simulink model "pacificpower360amxt"  (R2018b)
settings: Solver=VariableStepAuto  StartTime=0.0  StopTime=10  FixedStep=0.001  RelTol=1e-3
libraries: fl_lib x25, nesl_utility x19, powerlib_meascontrol x12, simulink x12
settings Model: Creator=opal  LastModifiedBy=mne4
settings SFSimCC: SimUseLocalCustomCode=off
settings RTWCC: RTWUseLocalCustomCode=off
settings CodeAppCC: StateflowObjectComments=on
settings SimscapeCC: SimscapeNormalizeSystem=off

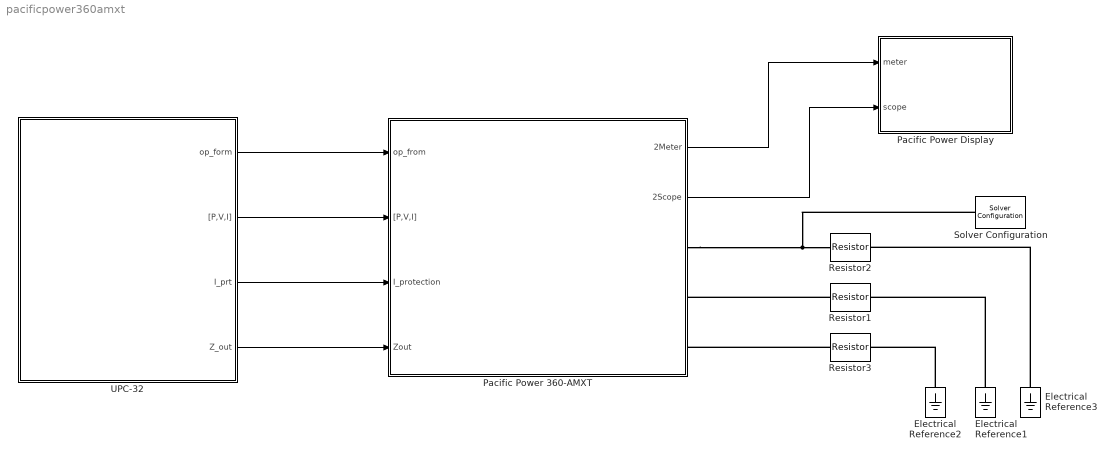
== system pacificpower360amxt ==
  Electrical Reference1 : fl_lib/Electrical/Electrical Elements/Electrical Reference
  Electrical Reference2 : fl_lib/Electrical/Electrical Elements/Electrical Reference
  Electrical Reference3 : fl_lib/Electrical/Electrical Elements/Electrical Reference
  Pacific Power 360-AMXT : Subsystem  mask{p_switch=1, VslewAC=5.000e+05, FslewAC=500.0, VslewDC=20000.0, IslewDC=1.000e+05, PslewDC=1.000e+06}
      mask prompts: p_switch "Enter 1 to turn ON, 0 to turn OFF NHR 9410"
      mask DialogControl DescTextVar Prompt: Pacific Power 360-AMXT (transformer coupled)
      mask DialogControl Container3 Prompt: Slew Rates
      mask DialogControl Control2 Prompt: AC Voltage slew rate [0-500000V/s]:
      mask DialogControl f Prompt: Frequency slew rate [0-500 /s]
      mask DialogControl Control3 Prompt: DC Voltage slew rate [0-20000V/s]:
      mask DialogControl Control4 Prompt: DC current slew rate [0-100000A/s]:
      mask DialogControl Control5 Prompt: DC power slew rate [0-1000000W/s]:
      mask Display: image('pacificpower360AMXT.png');
  Pacific Power Display : Subsystem
  Resistor1 : fl_lib/Electrical/Electrical Elements/Resistor  R=1.66 Ohm  i_specify=off  i_priority=None  i=0 A  i_nominal_specify=off  i_nominal_unit=A  i_nominal_value=1  v_specify=off  v_priority=None  v=0 V  v_nominal_specify=off  v_nominal_unit=V  v_nominal_value=1
  Resistor2 : fl_lib/Electrical/Electrical Elements/Resistor  R=1.66 Ohm  i_specify=off  i_priority=None  i=0 A  i_nominal_specify=off  i_nominal_unit=A  i_nominal_value=1  v_specify=off  v_priority=None  v=0 V  v_nominal_specify=off  v_nominal_unit=V  v_nominal_value=1
  Resistor3 : fl_lib/Electrical/Electrical Elements/Resistor  R=1.66 Ohm  i_specify=off  i_priority=None  i=0 A  i_nominal_specify=off  i_nominal_unit=A  i_nominal_value=1  v_specify=off  v_priority=None  v=0 V  v_nominal_specify=off  v_nominal_unit=V  v_nominal_value=1
  Solver Configuration : nesl_utility/Solver Configuration  PhysicalDomain=network_engine_domain  SubClassName=solver  LeftPortType=input  RightPortType=generic  Tones=[]  Harmonics=[]  SimulateNoise=off  Profile=off  UseLocalSampling=off  EnableSwitchedLinearOptims=on  FrequencyDomain=off  UseCCode=off  RelTol=0.001  AbsTol=1e-06  MinStep=1e-09  ToWorkspace=off  RevertToSquareIcSolve=off  NumHomotopyIterations=100  PhasorMode=off  PhasorModeNumHarmonics=1  DoDC=off  ResidualTolerance=1e-09  UseLocalSolver=on  LocalSolverChoice=NE_BACKWARD_EULER_ADVANCER  LocalSolverSampleTime=0.001  DoFixedCost=on  MaxNonlinIter=3  MaxModeIter=2  LinearAlgebra=Sparse  EquationFormulation=NE_TIME_EF  DelaysMemoryBudget=1024  AutomaticFiltering=off  FilteringTimeConstant=0.001  PartitionStorageMethod=AS_NEEDED  PartitionMemoryBudget=1024
  UPC-32 : Subsystem  mask{f=60, sel=1, form_sel=1, Vm11=100, Im11=10, Vm12=100, Im12=10, Vm13a=100, Vm13b=100, Vm13c=100, Ph13b=120, Ph13c=240, Im13=10, Vm21=100, Im21=0, Vm22=100, Im22=0, Vm23a=100, Vm23b=100, Vm23c=100, Ph23b=120, Ph23c=240, Im23=10, Zout=10, Iprt=0, Iprtlim=0, Tiprt=0}
      mask prompts: sel "Enter "1" for direct coupling, or "2" for transformner (2.0:1) coupling:"; form_sel "Enter "1" for 1-phase (Form-1), "2" for 2-phase (Form-2), "3" for 3-phase (Form-3):"; Iprt "Current protection (1: ON, 0: OFF):"; Iprtlim "Current protection limit:"; Tiprt "Current protection time:"
      mask DialogControl DescTextVar Prompt: UPC-32 (Universal Programmable Controller)
      mask DialogControl Control30 Prompt: Frequency (Hz) [20-5000Hz]:
      mask DialogControl Container12 Prompt: Direct Coupling
      mask DialogControl Container67 Prompt: Expand selected form and enter input parameters
      mask DialogControl Container66 Prompt: Form-1: 1-phase AC
      mask DialogControl Control311 Prompt: Voltage limit (Vrms l-n) [0-135V]:
      mask DialogControl Control29 Prompt: Current limit (Irms/phase) [0-48A]:
      mask DialogControl Container68 Prompt: Form-2: 2-phase AC
      mask DialogControl Control3_copy Prompt: Voltage limit (Vrms l-l) [0-270V]:
      mask DialogControl Control36 Prompt: Current limit (Irms/phase) [0-16A]:
      mask DialogControl Container69 Prompt: Form-3: 3-phase AC
      mask DialogControl Control331 Prompt: Voltage limit (Vrms l-n) [0-135V], Phase A:
      mask DialogControl Control31 Prompt: Voltage limit (Vrms l-n) [0-135V], Phase B:
      mask DialogControl Control32 Prompt: Voltage limit (Vrms l-n) [0-135V], Phase C:
      mask DialogControl Control33 Prompt: Phase A angle (degrees): 0
      mask DialogControl Control34 Prompt: Phase B angle (degrees):
      mask DialogControl Control35 Prompt: Phase C angle (degrees):
      mask DialogControl Control37 Prompt: Current limit (Irms/phase) [0-16A]:
      mask DialogControl Container12_copy Prompt: Transformer Coupling
      mask DialogControl Container67_copy Prompt: Expand selected form and enter input parameters
      mask DialogControl Container66_copy Prompt: Form-1: 1-phase AC
      mask DialogControl Control311_copy Prompt: Voltage limit (Vrms l-n) [0-273V]:
      mask DialogControl Control29_copy Prompt: Current limit (Irms/phase) [0-24A]:
      mask DialogControl Container68_copy Prompt: Form-2: 2-phase AC
      mask DialogControl Control3_copy_copy Prompt: Voltage limit (Vrms l-l) [0-546V]:
      mask DialogControl Control36_copy Prompt: Current limit (Irms/phase) [0-8A]:
      mask DialogControl Container69_copy Prompt: Form-3: 3-phase AC
      mask DialogControl Control331_copy Prompt: Voltage limit (Vrms l-n) [0-273V], Phase A:
      mask DialogControl Control31_copy Prompt: Voltage limit (Vrms l-n) [0-273V], Phase B:
      mask DialogControl Control32_copy Prompt: Voltage limit (Vrms l-n) [0-273V], Phase C:
      mask DialogControl Control33_copy Prompt: Phase A angle (degrees): 0
      mask DialogControl Control34_copy Prompt: Phase B angle (degrees):
      mask DialogControl Control35_copy Prompt: Phase C angle (degrees):
      mask DialogControl Control37_copy Prompt: Current limit (Irms/phase) [0-8A]:
      mask DialogControl Control27 Prompt: Output impedance
      mask Display: image('upc32.png');
  wires:
  UPC-32/1(op_form) -> Pacific Power 360-AMXT/1(op_from)
  UPC-32/2("[P,V,I]") -> Pacific Power 360-AMXT/2("[P,V,I]")
  UPC-32/3(I_prt) -> Pacific Power 360-AMXT/3(I_protection)
  UPC-32/4(Z_out) -> Pacific Power 360-AMXT/4(Zout)
  Pacific Power 360-AMXT/1(2Meter) -> Pacific Power Display/1(meter)
  Pacific Power 360-AMXT/2(2Scope) -> Pacific Power Display/2(scope)
  connections:
  Pacific Power 360-AMXT/RConn1 -- Solver Configuration/RConn1 -- Resistor2/LConn1
  Electrical Reference3/LConn1 -- Resistor2/RConn1
  Resistor1/LConn1 -- Pacific Power 360-AMXT/RConn2
  Resistor3/LConn1 -- Pacific Power 360-AMXT/RConn3
  Electrical Reference2/LConn1 -- Resistor3/RConn1
  Electrical Reference1/LConn1 -- Resistor1/RConn1

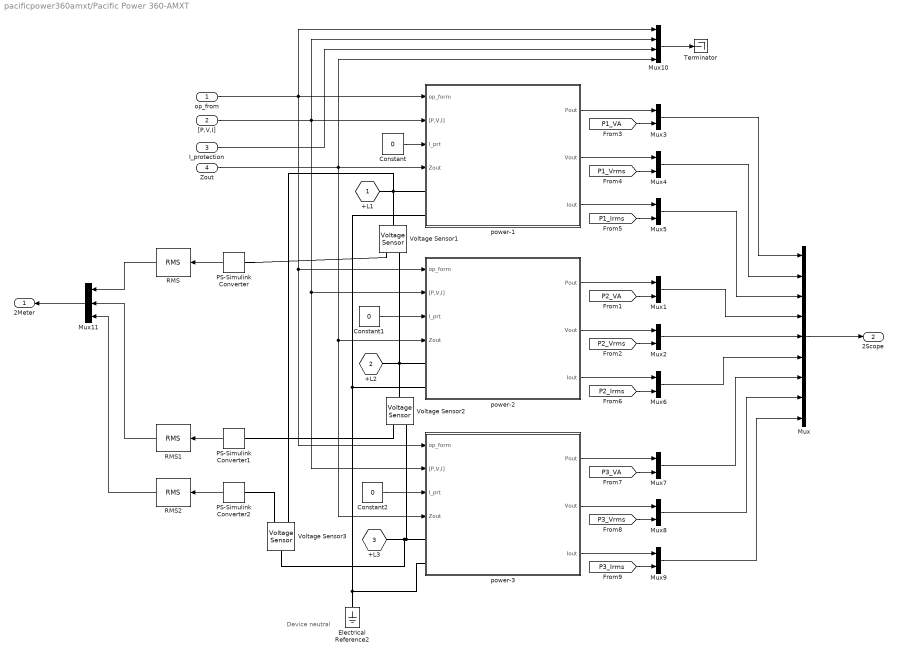
== system pacificpower360amxt/Pacific Power 360-AMXT ==
  note: Device neutral
  op_from : Inport
  "[P,V,I]" : Inport  Port=2
  I_protection : Inport  Port=3
  Zout : Inport  Port=4
  Constant : Constant  Value=0
  Constant1 : Constant  Value=0
  Constant2 : Constant  Value=0
  Electrical Reference2 : fl_lib/Electrical/Electrical Elements/Electrical Reference
  Mux : Mux  Inputs=9
  Mux{1..9} (9 alike) : Mux  Inputs=2
  Mux10 : Mux
  Mux11 : Mux  Inputs=3
  PS-Simulink Converter : nesl_utility/PS-Simulink Converter  PhysicalDomain=network_engine_domain  SubClassName=ps_output  LeftPortType=input  RightPortType=output  PseudoPeriodic=off  Frequencies=[]  Unit=1  AffineConversion=off
  PS-Simulink Converter1 : nesl_utility/PS-Simulink Converter  PhysicalDomain=network_engine_domain  SubClassName=ps_output  LeftPortType=input  RightPortType=output  PseudoPeriodic=off  Frequencies=[]  Unit=1  AffineConversion=off
  PS-Simulink Converter2 : nesl_utility/PS-Simulink Converter  PhysicalDomain=network_engine_domain  SubClassName=ps_output  LeftPortType=input  RightPortType=output  PseudoPeriodic=off  Frequencies=[]  Unit=1  AffineConversion=off
  RMS : powerlib_meascontrol/Measurements/RMS  TrueRMS=on  Freq=60  RMSInit=0  Ts=0
      settings: SourceProductName=Simscape Electrical
  RMS1 : powerlib_meascontrol/Measurements/RMS  TrueRMS=on  Freq=60  RMSInit=0  Ts=0
      settings: SourceProductName=Simscape Electrical
  RMS2 : powerlib_meascontrol/Measurements/RMS  TrueRMS=on  Freq=60  RMSInit=0  Ts=0
      settings: SourceProductName=Simscape Electrical
  Terminator : Terminator
  Voltage Sensor1 : fl_lib/Electrical/Electrical Sensors/Voltage Sensor
  Voltage Sensor2 : fl_lib/Electrical/Electrical Sensors/Voltage Sensor
  Voltage Sensor3 : fl_lib/Electrical/Electrical Sensors/Voltage Sensor
  power-1 : Subsystem
  power-2 : Subsystem
  power-3 : Subsystem
  +L1 : PMIOPort  Side=Right
  +L2 : PMIOPort  Port=2  Side=Right
  +L3 : PMIOPort  Port=3  Side=Right
  2Meter : Outport
  2Scope : Outport  Port=2
  wires:
  [P1_Irms] -> Mux5/2
  [P1_Vrms] -> Mux4/2
  [P1_VA] -> Mux3/2
  power-1/3(Iout) -> Mux5/1
  power-1/1(Pout) -> Mux3/1
  power-1/2(Vout) -> Mux4/1
  Zout/1 -> power-3/4(Zout), power-2/4(Zout), Mux10/4, power-1/4(Zout)
  I_protection/1 -> Mux10/3
  "[P,V,I]"/1 -> power-3/2("[P,V,I]"), power-2/2("[P,V,I]"), Mux10/2, power-1/2("[P,V,I]")
  Constant/1 -> power-1/3(I_prt)
  power-2/2(Vout) -> Mux2/1
  power-2/1(Pout) -> Mux1/1
  power-2/3(Iout) -> Mux6/1
  [P2_VA] -> Mux1/2
  [P2_Vrms] -> Mux2/2
  [P2_Irms] -> Mux6/2
  op_from/1 -> power-3/1(op_form), power-2/1(op_form), Mux10/1, power-1/1(op_form)
  Constant1/1 -> power-2/3(I_prt)
  [P3_Irms] -> Mux9/2
  [P3_Vrms] -> Mux8/2
  [P3_VA] -> Mux7/2
  power-3/3(Iout) -> Mux9/1
  power-3/1(Pout) -> Mux7/1
  power-3/2(Vout) -> Mux8/1
  Constant2/1 -> power-3/3(I_prt)
  Mux3/1 -> Mux/1
  Mux4/1 -> Mux/2
  Mux5/1 -> Mux/3
  Mux1/1 -> Mux/4
  Mux2/1 -> Mux/5
  Mux6/1 -> Mux/6
  Mux7/1 -> Mux/7
  Mux8/1 -> Mux/8
  Mux9/1 -> Mux/9
  Mux/1 -> 2Scope/1
  PS-Simulink Converter/1 -> RMS/1
  PS-Simulink Converter1/1 -> RMS1/1
  RMS/1 -> Mux11/1
  RMS1/1 -> Mux11/2
  Mux11/1 -> 2Meter/1
  Mux10/1 -> Terminator/1
  PS-Simulink Converter2/1 -> RMS2/1
  RMS2/1 -> Mux11/3
  connections:
  power-1/LConn2 -- power-2/LConn2 -- power-3/LConn2 -- Electrical Reference2/LConn1
  +L1/RConn1 -- Voltage Sensor3/RConn2 -- Voltage Sensor1/LConn1 -- power-1/LConn1
  +L2/RConn1 -- Voltage Sensor2/LConn1 -- Voltage Sensor1/RConn2 -- power-2/LConn1
  +L3/RConn1 -- power-3/LConn1 -- Voltage Sensor2/RConn2 -- Voltage Sensor3/LConn1
  PS-Simulink Converter/LConn1 -- Voltage Sensor1/RConn1
  PS-Simulink Converter1/LConn1 -- Voltage Sensor2/RConn1
  PS-Simulink Converter2/LConn1 -- Voltage Sensor3/RConn1

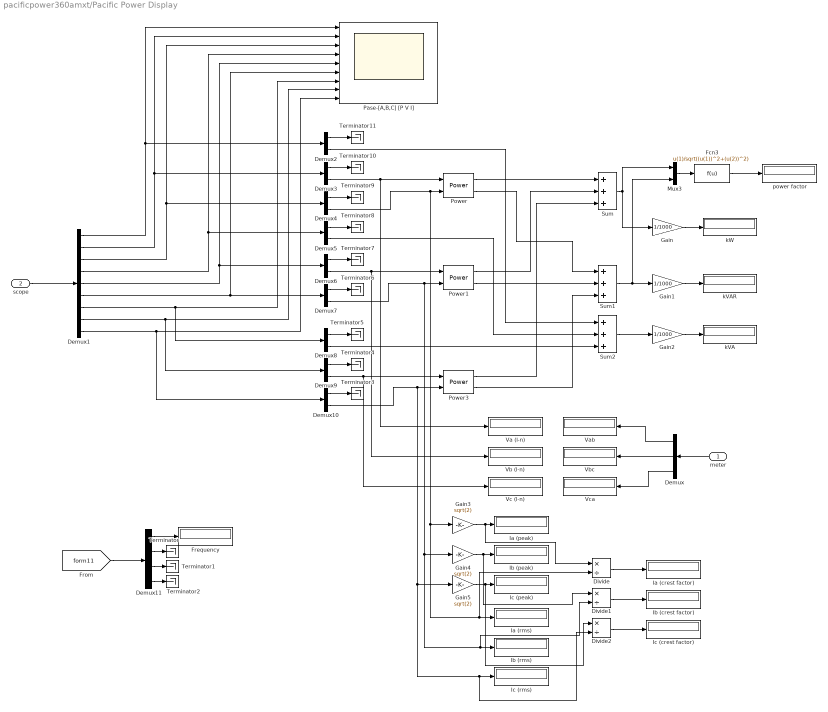
== system pacificpower360amxt/Pacific Power Display ==
  meter : Inport
  scope : Inport  Port=2
  Demux : Demux  Outputs=3
  Demux1 : Demux  Outputs=9
  Demux{2..10} (9 alike) : Demux  Outputs=2
  Demux11 : Demux
  Divide : Product  Inputs=*/
  Divide1 : Product  Inputs=*/
  Divide2 : Product  Inputs=*/
  Fcn3 : Fcn  Expr=u(1)/sqrt((u(1))^2+(u(2))^2)
  Frequency : Display
  Gain : Gain  Gain=1/1000
  Gain1 : Gain  Gain=1/1000
  Gain2 : Gain  Gain=1/1000
  Gain3 : Gain  Gain=sqrt(2)
  Gain4 : Gain  Gain=sqrt(2)
  Gain5 : Gain  Gain=sqrt(2)
  Ia (crest factor) : Display
      settings: Decimation=3
  Ia (peak) : Display
      settings: Decimation=3
  Ia (rms) : Display
      settings: Decimation=3
  Ib (crest factor) : Display
      settings: Decimation=3
  Ib (peak) : Display
      settings: Decimation=3
  Ib (rms) : Display
      settings: Decimation=3
  Ic (crest factor) : Display
      settings: Decimation=3
  Ic (peak) : Display
      settings: Decimation=3
  Ic (rms) : Display
      settings: Decimation=3
  Mux3 : Mux  Inputs=2
  Pase-[A,B,C] [P V I] : Scope  NumInputPorts=9
  Power : powerlib_meascontrol/Measurements/Power  Freq=60  Vinit=[1, 0]  Iinit=[1, 0]  Ts=0
      settings: SourceProductName=Simscape Electrical
  Power1 : powerlib_meascontrol/Measurements/Power  Freq=60  Vinit=[1, 0]  Iinit=[1, 0]  Ts=0
      settings: SourceProductName=Simscape Electrical
  Power3 : powerlib_meascontrol/Measurements/Power  Freq=60  Vinit=[1, 0]  Iinit=[1, 0]  Ts=0
      settings: SourceProductName=Simscape Electrical
  Sum : Sum  Inputs=+++
  Sum1 : Sum  Inputs=+++
  Sum2 : Sum  Inputs=+++
  Terminator{,1..11} (12 alike) : Terminator
  Va (l-n) : Display
      settings: Decimation=3
  Vab : Display
      settings: Decimation=3
  Vb (l-n) : Display
      settings: Decimation=3
  Vbc : Display
      settings: Decimation=3
  Vc (l-n) : Display
      settings: Decimation=3
  Vca : Display
      settings: Decimation=3
  kVA : Display
      settings: Decimation=3
  kVAR : Display
      settings: Decimation=3
  kW : Display
      settings: Decimation=3
  power factor : Display
  wires:
  meter/1 -> Demux/1
  scope/1 -> Demux1/1
  Demux1/6 -> Demux7/1, Pase-[A,B,C] [P V I]/6
  Demux1/2 -> Demux3/1, Pase-[A,B,C] [P V I]/2
  Demux1/4 -> Demux5/1, Pase-[A,B,C] [P V I]/4
  Demux1/1 -> Demux2/1, Pase-[A,B,C] [P V I]/1
  Demux1/8 -> Demux9/1, Pase-[A,B,C] [P V I]/8
  Demux1/3 -> Demux4/1, Pase-[A,B,C] [P V I]/3
  Demux1/7 -> Demux8/1, Pase-[A,B,C] [P V I]/7
  Demux1/5 -> Demux6/1, Pase-[A,B,C] [P V I]/5
  Demux1/9 -> Demux10/1, Pase-[A,B,C] [P V I]/9
  Demux6/2 -> Power1/1, Vb (l-n)/1
  Demux7/2 -> Divide1/2, Ib (rms)/1, Gain4/1, Power1/2
  Demux9/2 -> Power3/1, Vc (l-n)/1
  Demux10/2 -> Divide2/2, Ic (rms)/1, Gain5/1, Power3/2
  Power1/1 -> Sum/2
  Power3/1 -> Sum/3
  Power/1 -> Sum/1
  Sum/1 -> Gain/1, Mux3/1
  Gain/1 -> kW/1
  Gain1/1 -> kVAR/1
  Sum1/1 -> Mux3/2, Gain1/1
  Power/2 -> Sum1/1
  Power1/2 -> Sum1/2
  Power3/2 -> Sum1/3
  Mux3/1 -> Fcn3/1
  Fcn3/1 -> power factor/1
  Demux8/2 -> Sum2/3
  Demux5/2 -> Sum2/2
  Demux2/2 -> Sum2/1
  Sum2/1 -> Gain2/1
  Gain2/1 -> kVA/1
  Demux3/2 -> Power/1, Va (l-n)/1
  Demux/1 -> Vab/1
  Demux/2 -> Vbc/1
  Demux/3 -> Vca/1
  Gain3/1 -> Divide/1, Ia (peak)/1
  Gain4/1 -> Divide1/1, Ib (peak)/1
  Gain5/1 -> Divide2/1, Ic (peak)/1
  Divide/1 -> Ia (crest factor)/1
  Divide1/1 -> Ib (crest factor)/1
  Divide2/1 -> Ic (crest factor)/1
  Demux4/2 -> Divide/2, Ia (rms)/1, Gain3/1, Power/2
  [form11] -> Demux11/1
  Demux11/1 -> Frequency/1
  Demux11/2 -> Terminator/1
  Demux11/3 -> Terminator1/1
  Demux11/4 -> Terminator2/1
  Demux10/1 -> Terminator3/1
  Demux9/1 -> Terminator4/1
  Demux8/1 -> Terminator5/1
  Demux7/1 -> Terminator6/1
  Demux6/1 -> Terminator7/1
  Demux5/1 -> Terminator8/1
  Demux4/1 -> Terminator9/1
  Demux3/1 -> Terminator10/1
  Demux2/1 -> Terminator11/1

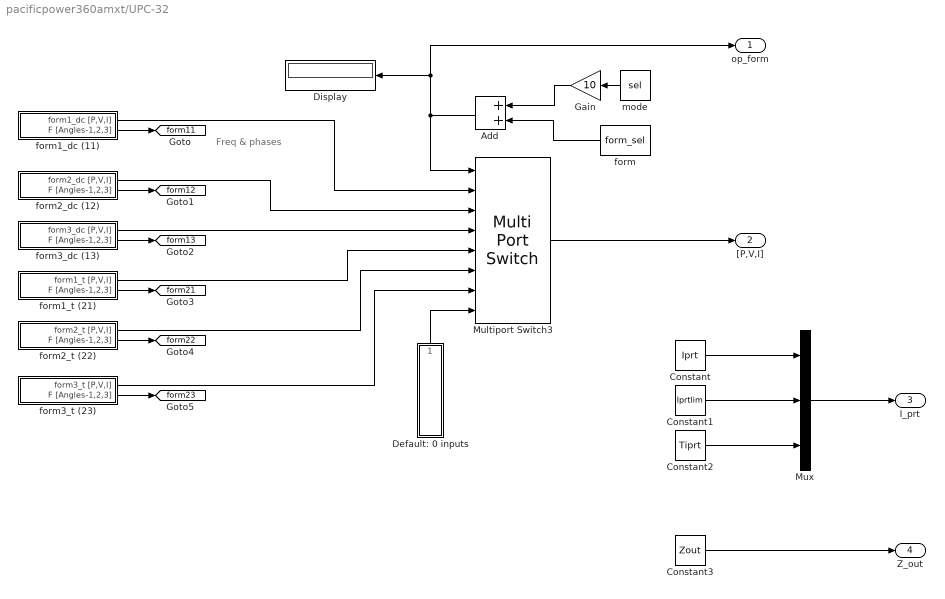
== system pacificpower360amxt/UPC-32 ==
  note: Freq & phases
  Add : Sum
  Constant : Constant  Value=Iprt
  Constant1 : Constant  Value=Iprtlim
  Constant2 : Constant  Value=Tiprt
  Constant3 : Constant  Value=Zout
  Default: 0 inputs : Subsystem
  Display : Display
  Gain : Gain  Gain=10
  Multiport Switch3 : MultiPortSwitch  DataPortOrder=Specify indices  Inputs=13  DataPortIndices={11,12,13,21,22,23}  DataPortForDefault=Additional data port  DiagnosticForDefault=None
  Mux : Mux  Inputs=3
  form : Constant  Value=form_sel
  form1_dc (11) : Subsystem
  form1_t (21) : Subsystem
  form2_dc (12) : Subsystem
  form2_t (22) : Subsystem
  form3_dc (13) : Subsystem
  form3_t (23) : Subsystem
  mode : Constant  Value=sel
  op_form : Outport
  "[P,V,I]" : Outport  Port=2
  I_prt : Outport  Port=3
  Z_out : Outport  Port=4
  tag scope: form11=global, form12=global, form13=global, form21=global, form22=global, form23=global
  wires:
  form3_t (23)/2(F [Angles-1,2,3]) -> [form23]
  form3_t (23)/1(form3_t [P,V,I]) -> Multiport Switch3/7
  Default: 0 inputs/1(form[1 2 3]) -> Multiport Switch3/8
  Gain/1 -> Add/1
  form2_t (22)/2(F [Angles-1,2,3]) -> [form22]
  form2_dc (12)/1(form2_dc [P,V,I]) -> Multiport Switch3/3
  form3_dc (13)/2(F [Angles-1,2,3]) -> [form13]
  form/1 -> Add/2
  form1_dc (11)/2(F [Angles-1,2,3]) -> [form11]
  form2_dc (12)/2(F [Angles-1,2,3]) -> [form12]
  form2_t (22)/1(form2_t [P,V,I]) -> Multiport Switch3/6
  mode/1 -> Gain/1
  form1_dc (11)/1(form1_dc [P,V,I]) -> Multiport Switch3/2
  form1_t (21)/1(form1_t [P,V,I]) -> Multiport Switch3/5
  form1_t (21)/2(F [Angles-1,2,3]) -> [form21]
  form3_dc (13)/1(form3_dc [P,V,I]) -> Multiport Switch3/4
  Add/1 -> op_form/1, Display/1, Multiport Switch3/1
  Multiport Switch3/1 -> "[P,V,I]"/1
  Constant/1 -> Mux/1
  Constant1/1 -> Mux/2
  Constant2/1 -> Mux/3
  Mux/1 -> I_prt/1
  Constant3/1 -> Z_out/1

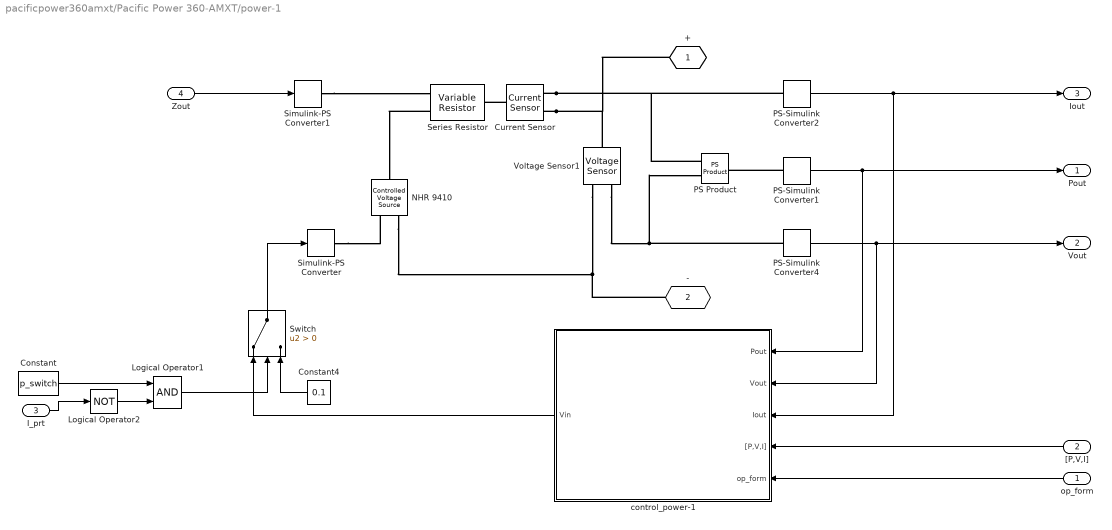
== system pacificpower360amxt/Pacific Power 360-AMXT/power-1 ==
  op_form : Inport
  "[P,V,I]" : Inport  Port=2
  I_prt : Inport  Port=3
  Zout : Inport  Port=4
  Constant : Constant  Value=p_switch
  Constant4 : Constant  Value=0.1
  Current Sensor : fl_lib/Electrical/Electrical Sensors/Current Sensor
  Logical Operator1 : Logic  AllPortsSameDT=off  OutDataTypeStr=boolean
  Logical Operator2 : Logic  Operator=NOT  AllPortsSameDT=off  OutDataTypeStr=boolean
  NHR 9410 : fl_lib/Electrical/Electrical Sources/Controlled Voltage Source
  PS Product : fl_lib/Physical Signals/Functions/PS Product
      settings: SourceProductName=Simscape
  PS-Simulink Converter1 : nesl_utility/PS-Simulink Converter  PhysicalDomain=network_engine_domain  SubClassName=ps_output  LeftPortType=input  RightPortType=output  PseudoPeriodic=off  Frequencies=[]  Unit=1  AffineConversion=off
  PS-Simulink Converter2 : nesl_utility/PS-Simulink Converter  PhysicalDomain=network_engine_domain  SubClassName=ps_output  LeftPortType=input  RightPortType=output  PseudoPeriodic=off  Frequencies=[]  Unit=1  AffineConversion=off
  PS-Simulink Converter4 : nesl_utility/PS-Simulink Converter  PhysicalDomain=network_engine_domain  SubClassName=ps_output  LeftPortType=input  RightPortType=output  PseudoPeriodic=off  Frequencies=[]  Unit=1  AffineConversion=off
  Series Resistor : fl_lib/Electrical/Electrical Elements/Variable Resistor  Rmin=0.0001 Ohm  i_specify=off  i_priority=None  i=0 A  i_nominal_specify=off  i_nominal_unit=A  i_nominal_value=1  v_specify=off  v_priority=None  v=0 V  v_nominal_specify=off  v_nominal_unit=V  v_nominal_value=1
  Simulink-PS Converter : nesl_utility/Simulink-PS Converter  PhysicalDomain=network_engine_domain  SubClassName=ps_input  LeftPortType=input  RightPortType=output  PseudoPeriodic=off  Frequencies=[]  NoiseDistribution=none  NoiseParameters=[]  Unit=1  AffineConversion=off  FilteringAndDerivatives=filter  SimscapeFilterOrder=1  InputFilterTimeConstant=0.001  UdotUserProvided=0
  Simulink-PS Converter1 : nesl_utility/Simulink-PS Converter  PhysicalDomain=network_engine_domain  SubClassName=ps_input  LeftPortType=input  RightPortType=output  PseudoPeriodic=off  Frequencies=[]  NoiseDistribution=none  NoiseParameters=[]  Unit=1  AffineConversion=off  FilteringAndDerivatives=filter  SimscapeFilterOrder=1  InputFilterTimeConstant=0.001  UdotUserProvided=0
  Switch : Switch  Criteria=u2 > Threshold  ZeroCross=off
  Voltage Sensor1 : fl_lib/Electrical/Electrical Sensors/Voltage Sensor
  control_power-1 : Subsystem
  + : PMIOPort  Tag=PMCPort  Side=Left
  - : PMIOPort  Tag=PMCPort  Port=2  Side=Left
  Pout : Outport
  Vout : Outport  Port=2
  Iout : Outport  Port=3
  wires:
  "[P,V,I]"/1 -> control_power-1/4("[P,V,I]")
  op_form/1 -> control_power-1/5(op_form)
  PS-Simulink Converter1/1 -> control_power-1/1(Pout), Pout/1
  PS-Simulink Converter4/1 -> control_power-1/2(Vout), Vout/1
  PS-Simulink Converter2/1 -> control_power-1/3(Iout), Iout/1
  Logical Operator1/1 -> Switch/2
  Constant4/1 -> Switch/3
  control_power-1/1(Vin) -> Switch/1
  Switch/1 -> Simulink-PS Converter/1
  Logical Operator2/1 -> Logical Operator1/2
  I_prt/1 -> Logical Operator2/1
  Constant/1 -> Logical Operator1/1
  Zout/1 -> Simulink-PS Converter1/1
  connections:
  PS-Simulink Converter4/LConn1 -- PS Product/LConn2 -- Voltage Sensor1/RConn1
  Voltage Sensor1/RConn2 -- -/RConn1 -- NHR 9410/RConn2
  Current Sensor/RConn1 -- PS-Simulink Converter2/LConn1 -- PS Product/LConn1
  Current Sensor/RConn2 -- +/RConn1 -- Voltage Sensor1/LConn1
  Simulink-PS Converter/RConn1 -- NHR 9410/RConn1
  Series Resistor/LConn2 -- NHR 9410/LConn1
  PS-Simulink Converter1/LConn1 -- PS Product/RConn1
  Simulink-PS Converter1/RConn1 -- Series Resistor/LConn1
  Current Sensor/LConn1 -- Series Resistor/RConn1

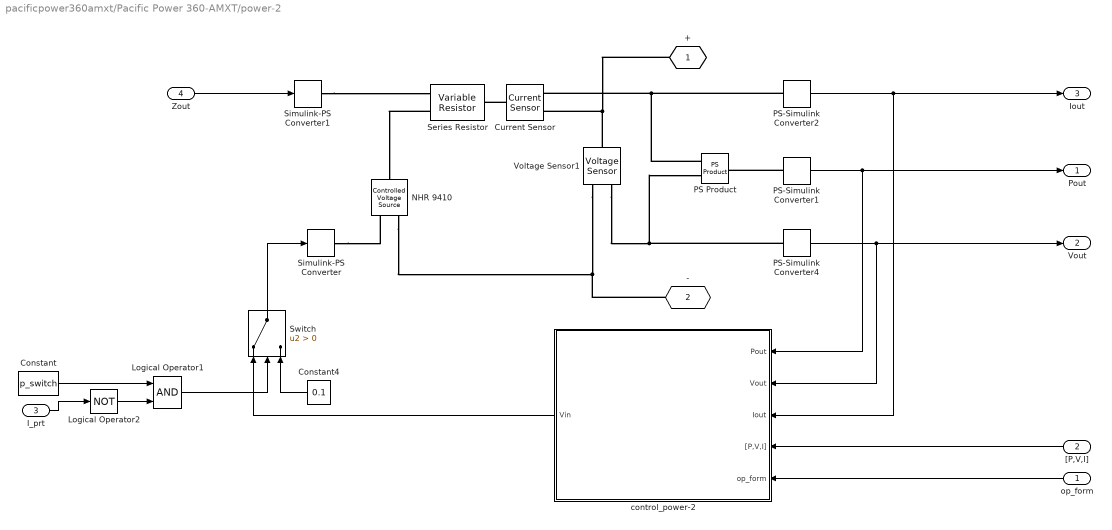
== system pacificpower360amxt/Pacific Power 360-AMXT/power-2 ==
  op_form : Inport
  "[P,V,I]" : Inport  Port=2
  I_prt : Inport  Port=3
  Zout : Inport  Port=4
  Constant : Constant  Value=p_switch
  Constant4 : Constant  Value=0.1
  Current Sensor : fl_lib/Electrical/Electrical Sensors/Current Sensor
  Logical Operator1 : Logic  AllPortsSameDT=off  OutDataTypeStr=boolean
  Logical Operator2 : Logic  Operator=NOT  AllPortsSameDT=off  OutDataTypeStr=boolean
  NHR 9410 : fl_lib/Electrical/Electrical Sources/Controlled Voltage Source
  PS Product : fl_lib/Physical Signals/Functions/PS Product
      settings: SourceProductName=Simscape
  PS-Simulink Converter1 : nesl_utility/PS-Simulink Converter  PhysicalDomain=network_engine_domain  SubClassName=ps_output  LeftPortType=input  RightPortType=output  PseudoPeriodic=off  Frequencies=[]  Unit=1  AffineConversion=off
  PS-Simulink Converter2 : nesl_utility/PS-Simulink Converter  PhysicalDomain=network_engine_domain  SubClassName=ps_output  LeftPortType=input  RightPortType=output  PseudoPeriodic=off  Frequencies=[]  Unit=1  AffineConversion=off
  PS-Simulink Converter4 : nesl_utility/PS-Simulink Converter  PhysicalDomain=network_engine_domain  SubClassName=ps_output  LeftPortType=input  RightPortType=output  PseudoPeriodic=off  Frequencies=[]  Unit=1  AffineConversion=off
  Series Resistor : fl_lib/Electrical/Electrical Elements/Variable Resistor  Rmin=0.0001 Ohm  i_specify=off  i_priority=None  i=0 A  i_nominal_specify=off  i_nominal_unit=A  i_nominal_value=1  v_specify=off  v_priority=None  v=0 V  v_nominal_specify=off  v_nominal_unit=V  v_nominal_value=1
  Simulink-PS Converter : nesl_utility/Simulink-PS Converter  PhysicalDomain=network_engine_domain  SubClassName=ps_input  LeftPortType=input  RightPortType=output  PseudoPeriodic=off  Frequencies=[]  NoiseDistribution=none  NoiseParameters=[]  Unit=1  AffineConversion=off  FilteringAndDerivatives=filter  SimscapeFilterOrder=1  InputFilterTimeConstant=0.001  UdotUserProvided=0
  Simulink-PS Converter1 : nesl_utility/Simulink-PS Converter  PhysicalDomain=network_engine_domain  SubClassName=ps_input  LeftPortType=input  RightPortType=output  PseudoPeriodic=off  Frequencies=[]  NoiseDistribution=none  NoiseParameters=[]  Unit=1  AffineConversion=off  FilteringAndDerivatives=filter  SimscapeFilterOrder=1  InputFilterTimeConstant=0.001  UdotUserProvided=0
  Switch : Switch  Criteria=u2 > Threshold  ZeroCross=off
  Voltage Sensor1 : fl_lib/Electrical/Electrical Sensors/Voltage Sensor
  control_power-2 : Subsystem
  + : PMIOPort  Tag=PMCPort  Side=Left
  - : PMIOPort  Tag=PMCPort  Port=2  Side=Left
  Pout : Outport
  Vout : Outport  Port=2
  Iout : Outport  Port=3
  wires:
  Zout/1 -> Simulink-PS Converter1/1
  Constant/1 -> Logical Operator1/1
  I_prt/1 -> Logical Operator2/1
  Logical Operator2/1 -> Logical Operator1/2
  Switch/1 -> Simulink-PS Converter/1
  control_power-2/1(Vin) -> Switch/1
  Constant4/1 -> Switch/3
  Logical Operator1/1 -> Switch/2
  PS-Simulink Converter2/1 -> Iout/1, control_power-2/3(Iout)
  PS-Simulink Converter4/1 -> Vout/1, control_power-2/2(Vout)
  PS-Simulink Converter1/1 -> Pout/1, control_power-2/1(Pout)
  op_form/1 -> control_power-2/5(op_form)
  "[P,V,I]"/1 -> control_power-2/4("[P,V,I]")
  connections:
  Current Sensor/LConn1 -- Series Resistor/RConn1
  Simulink-PS Converter1/RConn1 -- Series Resistor/LConn1
  PS-Simulink Converter1/LConn1 -- PS Product/RConn1
  Series Resistor/LConn2 -- NHR 9410/LConn1
  Simulink-PS Converter/RConn1 -- NHR 9410/RConn1
  Voltage Sensor1/LConn1 -- +/RConn1 -- Current Sensor/RConn2
  PS Product/LConn1 -- PS-Simulink Converter2/LConn1 -- Current Sensor/RConn1
  NHR 9410/RConn2 -- -/RConn1 -- Voltage Sensor1/RConn2
  Voltage Sensor1/RConn1 -- PS Product/LConn2 -- PS-Simulink Converter4/LConn1

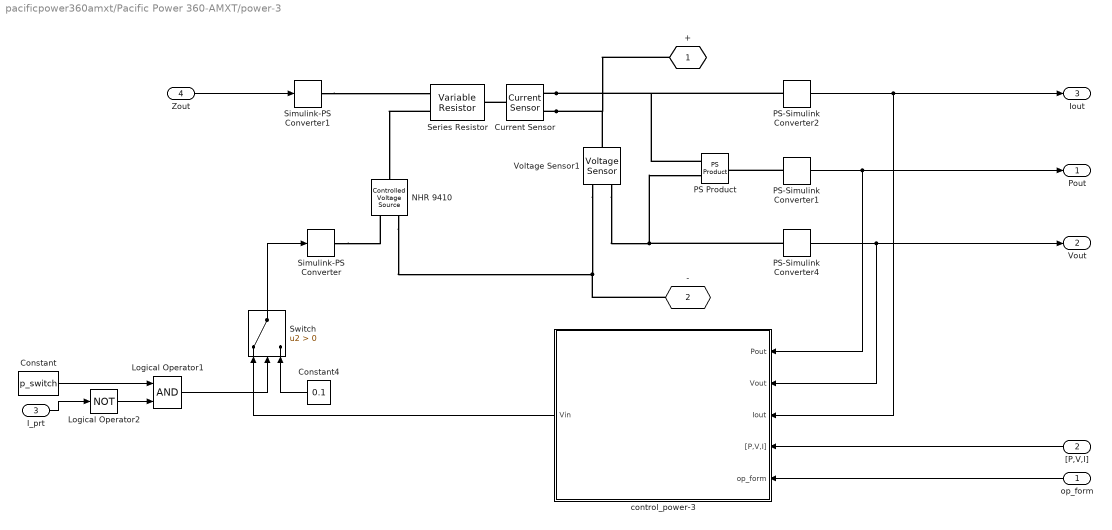
== system pacificpower360amxt/Pacific Power 360-AMXT/power-3 ==
  op_form : Inport
  "[P,V,I]" : Inport  Port=2
  I_prt : Inport  Port=3
  Zout : Inport  Port=4
  Constant : Constant  Value=p_switch
  Constant4 : Constant  Value=0.1
  Current Sensor : fl_lib/Electrical/Electrical Sensors/Current Sensor
  Logical Operator1 : Logic  AllPortsSameDT=off  OutDataTypeStr=boolean
  Logical Operator2 : Logic  Operator=NOT  AllPortsSameDT=off  OutDataTypeStr=boolean
  NHR 9410 : fl_lib/Electrical/Electrical Sources/Controlled Voltage Source
  PS Product : fl_lib/Physical Signals/Functions/PS Product
      settings: SourceProductName=Simscape
  PS-Simulink Converter1 : nesl_utility/PS-Simulink Converter  PhysicalDomain=network_engine_domain  SubClassName=ps_output  LeftPortType=input  RightPortType=output  PseudoPeriodic=off  Frequencies=[]  Unit=1  AffineConversion=off
  PS-Simulink Converter2 : nesl_utility/PS-Simulink Converter  PhysicalDomain=network_engine_domain  SubClassName=ps_output  LeftPortType=input  RightPortType=output  PseudoPeriodic=off  Frequencies=[]  Unit=1  AffineConversion=off
  PS-Simulink Converter4 : nesl_utility/PS-Simulink Converter  PhysicalDomain=network_engine_domain  SubClassName=ps_output  LeftPortType=input  RightPortType=output  PseudoPeriodic=off  Frequencies=[]  Unit=1  AffineConversion=off
  Series Resistor : fl_lib/Electrical/Electrical Elements/Variable Resistor  Rmin=0.0001 Ohm  i_specify=off  i_priority=None  i=0 A  i_nominal_specify=off  i_nominal_unit=A  i_nominal_value=1  v_specify=off  v_priority=None  v=0 V  v_nominal_specify=off  v_nominal_unit=V  v_nominal_value=1
  Simulink-PS Converter : nesl_utility/Simulink-PS Converter  PhysicalDomain=network_engine_domain  SubClassName=ps_input  LeftPortType=input  RightPortType=output  PseudoPeriodic=off  Frequencies=[]  NoiseDistribution=none  NoiseParameters=[]  Unit=1  AffineConversion=off  FilteringAndDerivatives=filter  SimscapeFilterOrder=1  InputFilterTimeConstant=0.001  UdotUserProvided=0
  Simulink-PS Converter1 : nesl_utility/Simulink-PS Converter  PhysicalDomain=network_engine_domain  SubClassName=ps_input  LeftPortType=input  RightPortType=output  PseudoPeriodic=off  Frequencies=[]  NoiseDistribution=none  NoiseParameters=[]  Unit=1  AffineConversion=off  FilteringAndDerivatives=filter  SimscapeFilterOrder=1  InputFilterTimeConstant=0.001  UdotUserProvided=0
  Switch : Switch  Criteria=u2 > Threshold  ZeroCross=off
  Voltage Sensor1 : fl_lib/Electrical/Electrical Sensors/Voltage Sensor
  control_power-3 : Subsystem
  + : PMIOPort  Tag=PMCPort  Side=Left
  - : PMIOPort  Tag=PMCPort  Port=2  Side=Left
  Pout : Outport
  Vout : Outport  Port=2
  Iout : Outport  Port=3
  wires:
  "[P,V,I]"/1 -> control_power-3/4("[P,V,I]")
  op_form/1 -> control_power-3/5(op_form)
  PS-Simulink Converter1/1 -> control_power-3/1(Pout), Pout/1
  PS-Simulink Converter4/1 -> control_power-3/2(Vout), Vout/1
  PS-Simulink Converter2/1 -> control_power-3/3(Iout), Iout/1
  Logical Operator1/1 -> Switch/2
  Constant4/1 -> Switch/3
  control_power-3/1(Vin) -> Switch/1
  Switch/1 -> Simulink-PS Converter/1
  Logical Operator2/1 -> Logical Operator1/2
  I_prt/1 -> Logical Operator2/1
  Constant/1 -> Logical Operator1/1
  Zout/1 -> Simulink-PS Converter1/1
  connections:
  PS-Simulink Converter4/LConn1 -- PS Product/LConn2 -- Voltage Sensor1/RConn1
  Voltage Sensor1/RConn2 -- -/RConn1 -- NHR 9410/RConn2
  Current Sensor/RConn1 -- PS-Simulink Converter2/LConn1 -- PS Product/LConn1
  Current Sensor/RConn2 -- +/RConn1 -- Voltage Sensor1/LConn1
  Simulink-PS Converter/RConn1 -- NHR 9410/RConn1
  Series Resistor/LConn2 -- NHR 9410/LConn1
  PS-Simulink Converter1/LConn1 -- PS Product/RConn1
  Simulink-PS Converter1/RConn1 -- Series Resistor/LConn1
  Current Sensor/LConn1 -- Series Resistor/RConn1

== system pacificpower360amxt/UPC-32/Default: 0 inputs ==
  form : Constant  Value=[0,0,0,0,0]
  form[1 2 3] : Outport
  wires:
  form/1 -> form[1 2 3]/1

== system pacificpower360amxt/UPC-32/form1_dc (11) ==
  Angle-1 : Constant  Value=0
  Frequency-1 : Constant  Value=f
  Mux3 : Mux  Inputs=3
  Mux4 : Mux
  form1_dc current : Constant  Value=Im11
  form1_dc power (VA) : Constant  Value=6000
  form1_dc voltage : Constant  Value=[Vm11,0,0]
  form1_dc [P,V,I] : Outport
  F [Angles-1,2,3] : Outport  Port=2
  wires:
  Mux4/1 -> F [Angles-1,2,3]/1
  Mux3/1 -> form1_dc [P,V,I]/1
  Frequency-1/1 -> Mux4/1
  form1_dc current/1 -> Mux3/3
  form1_dc voltage/1 -> Mux3/2
  form1_dc power (VA)/1 -> Mux3/1
  Angle-1/1 -> Mux4/2, Mux4/3, Mux4/4

== system pacificpower360amxt/UPC-32/form1_t (21) ==
  Angle-1 : Constant  Value=0
  Frequency-1 : Constant  Value=f
  Mux3 : Mux  Inputs=3
  Mux4 : Mux
  form1_t current : Constant  Value=Im21
  form1_t power (VA) : Constant  Value=6000
  form1_t voltage : Constant  Value=[Vm21,0,0]
  form1_t [P,V,I] : Outport
  F [Angles-1,2,3] : Outport  Port=2
  wires:
  Angle-1/1 -> Mux4/4, Mux4/3, Mux4/2
  form1_t power (VA)/1 -> Mux3/1
  form1_t voltage/1 -> Mux3/2
  form1_t current/1 -> Mux3/3
  Frequency-1/1 -> Mux4/1
  Mux3/1 -> form1_t [P,V,I]/1
  Mux4/1 -> F [Angles-1,2,3]/1

== system pacificpower360amxt/UPC-32/form2_dc (12) ==
  Angle-1 : Constant  Value=0
  Angle-2 : Constant  Value=180
  Frequency-1 : Constant  Value=f
  Mux3 : Mux  Inputs=3
  Mux4 : Mux
  form2_dc current : Constant  Value=Im12
  form2_dc power (VA) : Constant  Value=4500
  form2_dc voltage : Constant  Value=[Vm12/2,Vm12/2,0]
  form2_dc [P,V,I] : Outport
  F [Angles-1,2,3] : Outport  Port=2
  wires:
  form2_dc power (VA)/1 -> Mux3/1
  form2_dc voltage/1 -> Mux3/2
  form2_dc current/1 -> Mux3/3
  Frequency-1/1 -> Mux4/1
  Mux3/1 -> form2_dc [P,V,I]/1
  Mux4/1 -> F [Angles-1,2,3]/1
  Angle-2/1 -> Mux4/3
  Angle-1/1 -> Mux4/4, Mux4/2

== system pacificpower360amxt/UPC-32/form2_t (22) ==
  Angle-1 : Constant  Value=0
  Angle-2 : Constant  Value=180
  Frequency-1 : Constant  Value=f
  Mux3 : Mux  Inputs=3
  Mux4 : Mux
  form2_t current : Constant  Value=Im22
  form2_t power (VA) : Constant  Value=4500
  form2_t voltage : Constant  Value=[Vm22/2,Vm22/2,0]
  form2_t [P,V,I] : Outport
  F [Angles-1,2,3] : Outport  Port=2
  wires:
  Angle-1/1 -> Mux4/2, Mux4/4
  Angle-2/1 -> Mux4/3
  Mux4/1 -> F [Angles-1,2,3]/1
  Mux3/1 -> form2_t [P,V,I]/1
  Frequency-1/1 -> Mux4/1
  form2_t current/1 -> Mux3/3
  form2_t voltage/1 -> Mux3/2
  form2_t power (VA)/1 -> Mux3/1

== system pacificpower360amxt/UPC-32/form3_dc (13) ==
  Angle-1 : Constant  Value=0
  Angle-2 : Constant  Value=Ph13b
  Angle-3 : Constant  Value=Ph13c
  Frequency-1 : Constant  Value=f
  Mux3 : Mux  Inputs=3
  Mux4 : Mux
  form3_dc current : Constant  Value=Im13
  form3_dc power (VA) : Constant  Value=6000
  form3_dc voltage : Constant  Value=[Vm13a,Vm13b,Vm13c]
  form3_dc [P,V,I] : Outport
  F [Angles-1,2,3] : Outport  Port=2
  wires:
  Angle-1/1 -> Mux4/2
  Mux4/1 -> F [Angles-1,2,3]/1
  Mux3/1 -> form3_dc [P,V,I]/1
  Frequency-1/1 -> Mux4/1
  form3_dc current/1 -> Mux3/3
  form3_dc voltage/1 -> Mux3/2
  form3_dc power (VA)/1 -> Mux3/1
  Angle-2/1 -> Mux4/3
  Angle-3/1 -> Mux4/4

== system pacificpower360amxt/UPC-32/form3_t (23) ==
  Angle-1 : Constant  Value=0
  Angle-2 : Constant  Value=Ph23b
  Angle-3 : Constant  Value=Ph23c
  Frequency-1 : Constant  Value=f
  Mux3 : Mux  Inputs=3
  Mux4 : Mux
  form3_t current : Constant  Value=Im23
  form3_t power (VA) : Constant  Value=6000
  form3_t voltage : Constant  Value=[Vm23a,Vm23b,Vm23c]
  form3_t [P,V,I] : Outport
  F [Angles-1,2,3] : Outport  Port=2
  wires:
  Angle-3/1 -> Mux4/4
  Angle-2/1 -> Mux4/3
  form3_t power (VA)/1 -> Mux3/1
  form3_t voltage/1 -> Mux3/2
  form3_t current/1 -> Mux3/3
  Frequency-1/1 -> Mux4/1
  Mux3/1 -> form3_t [P,V,I]/1
  Mux4/1 -> F [Angles-1,2,3]/1
  Angle-1/1 -> Mux4/2

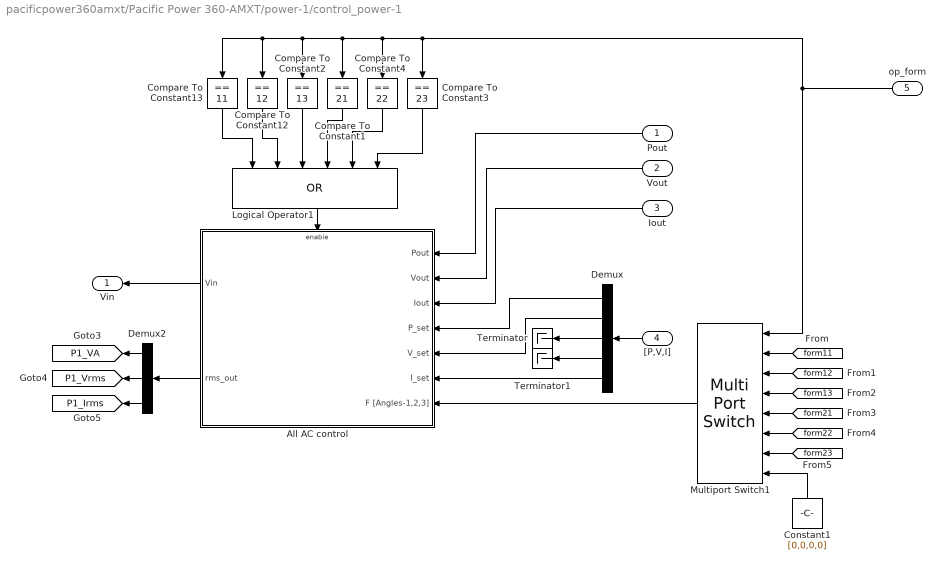
== system pacificpower360amxt/Pacific Power 360-AMXT/power-1/control_power-1 ==
  Pout : Inport
  Vout : Inport  Port=2
  Iout : Inport  Port=3
  "[P,V,I]" : Inport  Port=4
  op_form : Inport  Port=5
  All AC control : Subsystem
      settings: MinAlgLoopOccurrences=on
  Compare To Constant1 : simulink/Logic and Bit Operations/Compare To Constant  relop===  const=21  OutDataTypeStr=boolean
  Compare To Constant12 : simulink/Logic and Bit Operations/Compare To Constant  relop===  const=12  OutDataTypeStr=boolean
  Compare To Constant13 : simulink/Logic and Bit Operations/Compare To Constant  relop===  const=11  OutDataTypeStr=boolean
  Compare To Constant2 : simulink/Logic and Bit Operations/Compare To Constant  relop===  const=13  OutDataTypeStr=boolean
  Compare To Constant3 : simulink/Logic and Bit Operations/Compare To Constant  relop===  const=23  OutDataTypeStr=boolean
  Compare To Constant4 : simulink/Logic and Bit Operations/Compare To Constant  relop===  const=22  OutDataTypeStr=boolean
  Constant1 : Constant  Value=[0,0,0,0]
  Demux : Demux  Outputs=5
  Demux2 : Demux  Outputs=3
  Logical Operator1 : Logic  Operator=OR  Inputs=6  AllPortsSameDT=off  OutDataTypeStr=boolean
  Multiport Switch1 : MultiPortSwitch  DataPortOrder=Specify indices  Inputs=13  DataPortIndices={11,12,13,21,22,23}  DataPortForDefault=Additional data port  DiagnosticForDefault=None
  Terminator : Terminator
  Terminator1 : Terminator
  Vin : Outport
  tag scope: P1_Irms=global, P1_VA=global, P1_Vrms=global
  wires:
  All AC control/1(Vin) -> Vin/1
  "[P,V,I]"/1 -> Demux/1
  Vout/1 -> All AC control/2(Vout)
  Demux2/2 -> [P1_Vrms]
  Demux2/3 -> [P1_Irms]
  Demux2/1 -> [P1_VA]
  Iout/1 -> All AC control/3(Iout)
  Pout/1 -> All AC control/1(Pout)
  Logical Operator1/1 -> All AC control/Enable
  All AC control/2(rms_out) -> Demux2/1
  Multiport Switch1/1 -> All AC control/7(F [Angles-1,2,3])
  op_form/1 -> Compare To Constant3/1, Compare To Constant4/1, Compare To Constant1/1, Compare To Constant2/1, Compare To Constant12/1, Compare To Constant13/1, Multiport Switch1/1
  Constant1/1 -> Multiport Switch1/8
  [form11] -> Multiport Switch1/2
  [form23] -> Multiport Switch1/7
  [form22] -> Multiport Switch1/6
  [form21] -> Multiport Switch1/5
  [form13] -> Multiport Switch1/4
  [form12] -> Multiport Switch1/3
  Compare To Constant3/1 -> Logical Operator1/6
  Compare To Constant4/1 -> Logical Operator1/5
  Compare To Constant1/1 -> Logical Operator1/4
  Compare To Constant2/1 -> Logical Operator1/3
  Compare To Constant12/1 -> Logical Operator1/2
  Compare To Constant13/1 -> Logical Operator1/1
  Demux/1 -> All AC control/4(P_set)
  Demux/2 -> All AC control/5(V_set)
  Demux/5 -> All AC control/6(I_set)
  Demux/3 -> Terminator/1
  Demux/4 -> Terminator1/1

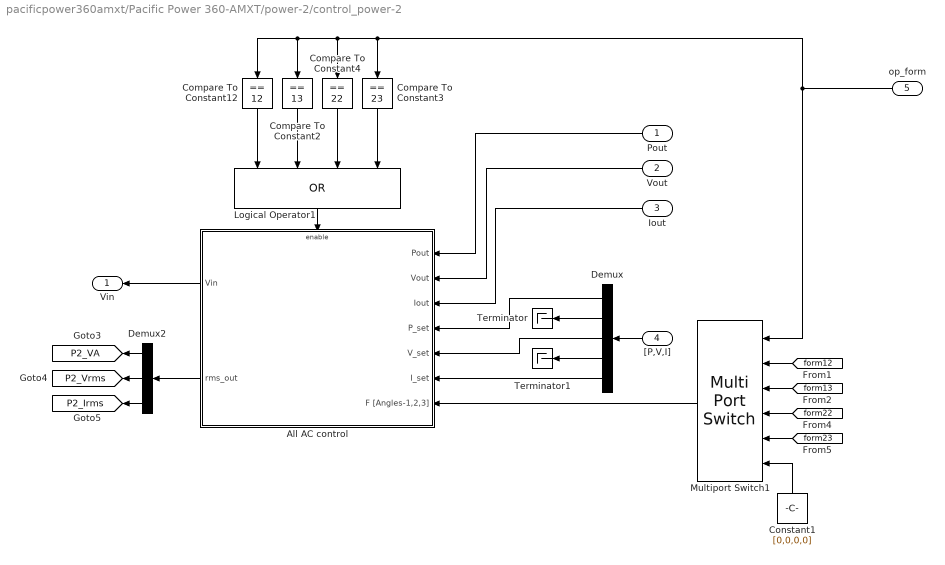
== system pacificpower360amxt/Pacific Power 360-AMXT/power-2/control_power-2 ==
  Pout : Inport
  Vout : Inport  Port=2
  Iout : Inport  Port=3
  "[P,V,I]" : Inport  Port=4
  op_form : Inport  Port=5
  All AC control : Subsystem
      settings: MinAlgLoopOccurrences=on
  Compare To Constant12 : simulink/Logic and Bit Operations/Compare To Constant  relop===  const=12  OutDataTypeStr=boolean
  Compare To Constant2 : simulink/Logic and Bit Operations/Compare To Constant  relop===  const=13  OutDataTypeStr=boolean
  Compare To Constant3 : simulink/Logic and Bit Operations/Compare To Constant  relop===  const=23  OutDataTypeStr=boolean
  Compare To Constant4 : simulink/Logic and Bit Operations/Compare To Constant  relop===  const=22  OutDataTypeStr=boolean
  Constant1 : Constant  Value=[0,0,0,0]
  Demux : Demux  Outputs=5
  Demux2 : Demux  Outputs=3
  Logical Operator1 : Logic  Operator=OR  Inputs=4  AllPortsSameDT=off  OutDataTypeStr=boolean
  Multiport Switch1 : MultiPortSwitch  DataPortOrder=Specify indices  Inputs=13  DataPortIndices={12,13,22,23}  DataPortForDefault=Additional data port  DiagnosticForDefault=None
  Terminator : Terminator
  Terminator1 : Terminator
  Vin : Outport
  tag scope: P2_Irms=global, P2_VA=global, P2_Vrms=global
  wires:
  Demux/4 -> Terminator1/1
  Demux/5 -> All AC control/6(I_set)
  Demux/1 -> All AC control/4(P_set)
  op_form/1 -> Multiport Switch1/1, Compare To Constant12/1, Compare To Constant2/1, Compare To Constant4/1, Compare To Constant3/1
  Multiport Switch1/1 -> All AC control/7(F [Angles-1,2,3])
  All AC control/2(rms_out) -> Demux2/1
  Logical Operator1/1 -> All AC control/Enable
  Pout/1 -> All AC control/1(Pout)
  Iout/1 -> All AC control/3(Iout)
  Demux2/1 -> [P2_VA]
  Demux2/3 -> [P2_Irms]
  Demux2/2 -> [P2_Vrms]
  Vout/1 -> All AC control/2(Vout)
  "[P,V,I]"/1 -> Demux/1
  All AC control/1(Vin) -> Vin/1
  Compare To Constant12/1 -> Logical Operator1/1
  Compare To Constant2/1 -> Logical Operator1/2
  Compare To Constant4/1 -> Logical Operator1/3
  Compare To Constant3/1 -> Logical Operator1/4
  [form12] -> Multiport Switch1/2
  [form13] -> Multiport Switch1/3
  [form22] -> Multiport Switch1/4
  [form23] -> Multiport Switch1/5
  Constant1/1 -> Multiport Switch1/6
  Demux/2 -> Terminator/1
  Demux/3 -> All AC control/5(V_set)

== system pacificpower360amxt/Pacific Power 360-AMXT/power-3/control_power-3 ==
  Pout : Inport
  Vout : Inport  Port=2
  Iout : Inport  Port=3
  "[P,V,I]" : Inport  Port=4
  op_form : Inport  Port=5
  Compare To Constant2 : simulink/Logic and Bit Operations/Compare To Constant  relop===  const=13  OutDataTypeStr=boolean
  Compare To Constant3 : simulink/Logic and Bit Operations/Compare To Constant  relop===  const=23  OutDataTypeStr=boolean
  Constant1 : Constant  Value=[0,0,0,0]
  Demux : Demux  Outputs=5
  Demux2 : Demux  Outputs=3
  Logical Operator1 : Logic  Operator=OR  AllPortsSameDT=off  OutDataTypeStr=boolean
  Multiport Switch1 : MultiPortSwitch  DataPortOrder=Specify indices  Inputs=13  DataPortIndices={13,23}  DataPortForDefault=Additional data port  DiagnosticForDefault=None
  Terminator : Terminator
  Terminator1 : Terminator
  conrol : Subsystem
      settings: MinAlgLoopOccurrences=on
  Vin : Outport
  tag scope: P3_Irms=global, P3_VA=global, P3_Vrms=global
  wires:
  Demux/2 -> Terminator/1
  [form23] -> Multiport Switch1/3
  [form13] -> Multiport Switch1/2
  Compare To Constant3/1 -> Logical Operator1/2
  Compare To Constant2/1 -> Logical Operator1/1
  conrol/1(Vin) -> Vin/1
  "[P,V,I]"/1 -> Demux/1
  Vout/1 -> conrol/2(Vout)
  Demux2/2 -> [P3_Vrms]
  Demux2/3 -> [P3_Irms]
  Demux2/1 -> [P3_VA]
  Iout/1 -> conrol/3(Iout)
  Pout/1 -> conrol/1(Pout)
  Logical Operator1/1 -> conrol/Enable
  conrol/2(rms_out) -> Demux2/1
  Multiport Switch1/1 -> conrol/7(F [Angles-1,2,3])
  op_form/1 -> Compare To Constant3/1, Compare To Constant2/1, Multiport Switch1/1
  Demux/1 -> conrol/4(P_set)
  Demux/5 -> conrol/6(I_set)
  Demux/3 -> Terminator1/1
  Demux/4 -> conrol/5(V_set)
  Constant1/1 -> Multiport Switch1/4

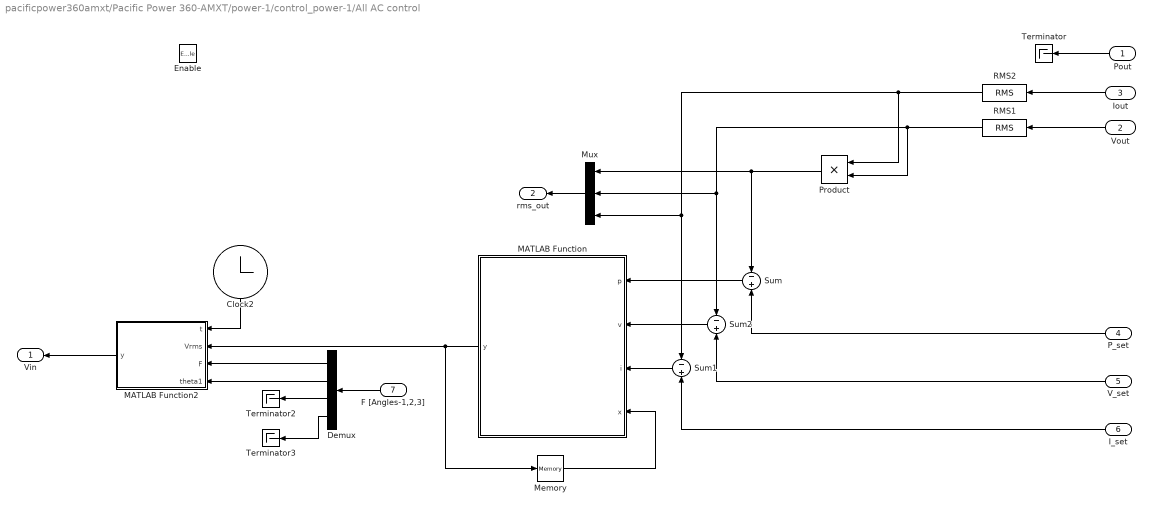
== system pacificpower360amxt/Pacific Power 360-AMXT/power-1/control_power-1/All AC control ==
  Pout : Inport
  Vout : Inport  Port=2
  Iout : Inport  Port=3
  P_set : Inport  Port=4
  V_set : Inport  Port=5
  I_set : Inport  Port=6
  F [Angles-1,2,3] : Inport  Port=7
  Enable : EnablePort
  Clock2 : Clock
  Demux : Demux
  MATLAB Function : MATLAB Function  TreatAsAtomicUnit=on
  MATLAB Function2 : MATLAB Function  TreatAsAtomicUnit=on
  Memory : Memory
  Mux : Mux  Inputs=3
  Product : Product
  RMS1 : powerlib_meascontrol/Measurements/RMS  TrueRMS=on  Freq=60  RMSInit=0  Ts=0
      settings: SourceProductName=Simscape Electrical
  RMS2 : powerlib_meascontrol/Measurements/RMS  TrueRMS=on  Freq=60  RMSInit=0  Ts=0
      settings: SourceProductName=Simscape Electrical
  Sum : Sum  Inputs=-+
  Sum1 : Sum  Inputs=-+
  Sum2 : Sum  Inputs=-+
  Terminator : Terminator
  Terminator2 : Terminator
  Terminator3 : Terminator
  Vin : Outport
  rms_out : Outport  Port=2
  wires:
  Vout/1 -> RMS1/1
  MATLAB Function/1(y) -> MATLAB Function2/2(Vrms), Memory/1
  Iout/1 -> RMS2/1
  Pout/1 -> Terminator/1
  Sum/1 -> MATLAB Function/1(p)
  Sum2/1 -> MATLAB Function/2(v)
  Sum1/1 -> MATLAB Function/3(i)
  I_set/1 -> Sum1/2
  P_set/1 -> Sum/2
  RMS1/1 -> Product/2, Mux/2, Sum2/1
  RMS2/1 -> Product/1, Mux/3, Sum1/1
  Memory/1 -> MATLAB Function/4(x)
  Clock2/1 -> MATLAB Function2/1(t)
  MATLAB Function2/1(y) -> Vin/1
  Product/1 -> Mux/1, Sum/1
  Mux/1 -> rms_out/1
  F [Angles-1,2,3]/1 -> Demux/1
  V_set/1 -> Sum2/2
  Demux/1 -> MATLAB Function2/3(F)
  Demux/3 -> Terminator2/1
  Demux/4 -> Terminator3/1
  Demux/2 -> MATLAB Function2/4(theta1)

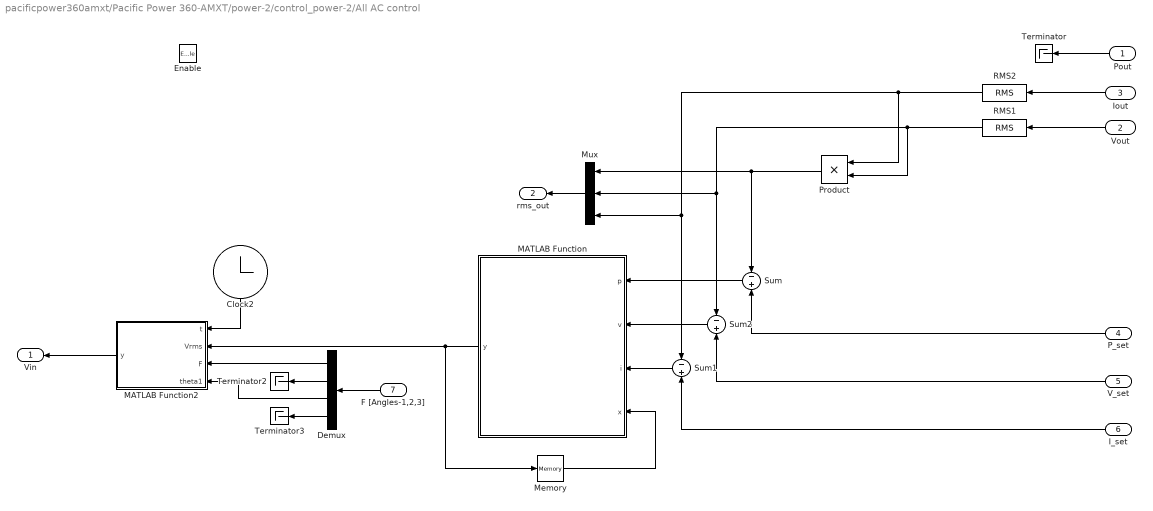
== system pacificpower360amxt/Pacific Power 360-AMXT/power-2/control_power-2/All AC control ==
  Pout : Inport
  Vout : Inport  Port=2
  Iout : Inport  Port=3
  P_set : Inport  Port=4
  V_set : Inport  Port=5
  I_set : Inport  Port=6
  F [Angles-1,2,3] : Inport  Port=7
  Enable : EnablePort
  Clock2 : Clock
  Demux : Demux
  MATLAB Function : MATLAB Function  TreatAsAtomicUnit=on
  MATLAB Function2 : MATLAB Function  TreatAsAtomicUnit=on
  Memory : Memory
  Mux : Mux  Inputs=3
  Product : Product
  RMS1 : powerlib_meascontrol/Measurements/RMS  TrueRMS=on  Freq=60  RMSInit=0  Ts=0
      settings: SourceProductName=Simscape Electrical
  RMS2 : powerlib_meascontrol/Measurements/RMS  TrueRMS=on  Freq=60  RMSInit=0  Ts=0
      settings: SourceProductName=Simscape Electrical
  Sum : Sum  Inputs=-+
  Sum1 : Sum  Inputs=-+
  Sum2 : Sum  Inputs=-+
  Terminator : Terminator
  Terminator2 : Terminator
  Terminator3 : Terminator
  Vin : Outport
  rms_out : Outport  Port=2
  wires:
  Demux/4 -> Terminator3/1
  Demux/1 -> MATLAB Function2/3(F)
  V_set/1 -> Sum2/2
  F [Angles-1,2,3]/1 -> Demux/1
  Mux/1 -> rms_out/1
  Product/1 -> Sum/1, Mux/1
  MATLAB Function2/1(y) -> Vin/1
  Clock2/1 -> MATLAB Function2/1(t)
  Memory/1 -> MATLAB Function/4(x)
  RMS2/1 -> Sum1/1, Mux/3, Product/1
  RMS1/1 -> Sum2/1, Mux/2, Product/2
  P_set/1 -> Sum/2
  I_set/1 -> Sum1/2
  Sum1/1 -> MATLAB Function/3(i)
  Sum2/1 -> MATLAB Function/2(v)
  Sum/1 -> MATLAB Function/1(p)
  Pout/1 -> Terminator/1
  Iout/1 -> RMS2/1
  MATLAB Function/1(y) -> Memory/1, MATLAB Function2/2(Vrms)
  Vout/1 -> RMS1/1
  Demux/2 -> Terminator2/1
  Demux/3 -> MATLAB Function2/4(theta1)

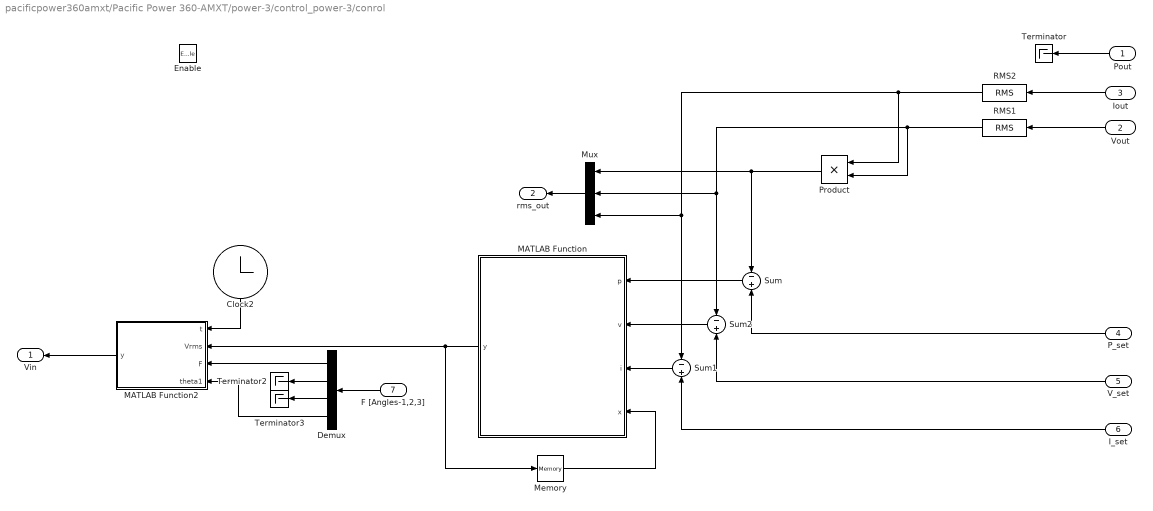
== system pacificpower360amxt/Pacific Power 360-AMXT/power-3/control_power-3/conrol ==
  Pout : Inport
  Vout : Inport  Port=2
  Iout : Inport  Port=3
  P_set : Inport  Port=4
  V_set : Inport  Port=5
  I_set : Inport  Port=6
  F [Angles-1,2,3] : Inport  Port=7
  Enable : EnablePort
  Clock2 : Clock
  Demux : Demux
  MATLAB Function : MATLAB Function  TreatAsAtomicUnit=on
  MATLAB Function2 : MATLAB Function  TreatAsAtomicUnit=on
  Memory : Memory
  Mux : Mux  Inputs=3
  Product : Product
  RMS1 : powerlib_meascontrol/Measurements/RMS  TrueRMS=on  Freq=60  RMSInit=0  Ts=0
      settings: SourceProductName=Simscape Electrical
  RMS2 : powerlib_meascontrol/Measurements/RMS  TrueRMS=on  Freq=60  RMSInit=0  Ts=0
      settings: SourceProductName=Simscape Electrical
  Sum : Sum  Inputs=-+
  Sum1 : Sum  Inputs=-+
  Sum2 : Sum  Inputs=-+
  Terminator : Terminator
  Terminator2 : Terminator
  Terminator3 : Terminator
  Vin : Outport
  rms_out : Outport  Port=2
  wires:
  Demux/2 -> Terminator2/1
  Vout/1 -> RMS1/1
  MATLAB Function/1(y) -> MATLAB Function2/2(Vrms), Memory/1
  Iout/1 -> RMS2/1
  Pout/1 -> Terminator/1
  Sum/1 -> MATLAB Function/1(p)
  Sum2/1 -> MATLAB Function/2(v)
  Sum1/1 -> MATLAB Function/3(i)
  I_set/1 -> Sum1/2
  P_set/1 -> Sum/2
  RMS1/1 -> Product/2, Mux/2, Sum2/1
  RMS2/1 -> Product/1, Mux/3, Sum1/1
  Memory/1 -> MATLAB Function/4(x)
  Clock2/1 -> MATLAB Function2/1(t)
  MATLAB Function2/1(y) -> Vin/1
  Product/1 -> Mux/1, Sum/1
  Mux/1 -> rms_out/1
  F [Angles-1,2,3]/1 -> Demux/1
  V_set/1 -> Sum2/2
  Demux/1 -> MATLAB Function2/3(F)
  Demux/3 -> Terminator3/1
  Demux/4 -> MATLAB Function2/4(theta1)

== matlab function pacificpower360amxt/Pacific Power 360-AMXT/power-1/control_power-1/All AC control/MATLAB Function ==
  data: p input; v input; y output; i input; x input
function y = fcn(p,v,i,x)
tol=1e-3;
gain=1e-4;
Ts=1e-3;
if p<=(-tol)
    y=x-(gain/Ts);
elseif i<=(-tol)
    y=x-(gain/Ts);
elseif v<=(-tol)
    y=x-(gain/Ts);
elseif v>tol;
    y=x+(gain/Ts);
else
    y=0;
end

== matlab function pacificpower360amxt/Pacific Power 360-AMXT/power-2/control_power-2/All AC control/MATLAB Function ==
  data: p input; v input; y output; i input; x input
function y = fcn(p,v,i,x)
tol=1e-3;
gain=1e-4;
Ts=1e-3;
if p<=(-tol)
    y=x-(gain/Ts);
elseif i<=(-tol)
    y=x-(gain/Ts);
elseif v<=(-tol)
    y=x-(gain/Ts);
elseif v>tol;
    y=x+(gain/Ts);
else
    y=0;
end

== matlab function pacificpower360amxt/Pacific Power 360-AMXT/power-1/control_power-1/All AC control/MATLAB Function2 ==
  data: t input; y output; Vrms input; F input; theta1 input
function y = fcn(t,Vrms,F,theta1)
y = sqrt(2)*Vrms*sin(2*pi*F*t + theta1*pi/180);

== matlab function pacificpower360amxt/Pacific Power 360-AMXT/power-2/control_power-2/All AC control/MATLAB Function2 ==
  data: t input; y output; Vrms input; F input; theta1 input
function y = fcn(t,Vrms,F,theta1)
y = sqrt(2)*Vrms*sin(2*pi*F*t + theta1*pi/180);

== matlab function pacificpower360amxt/Pacific Power 360-AMXT/power-3/control_power-3/conrol/MATLAB Function ==
  data: p input; v input; y output; i input; x input
function y = fcn(p,v,i,x)
tol=1e-3;
gain=1e-4;
Ts=1e-3;
if p<=(-tol)
    y=x-(gain/Ts);
elseif i<=(-tol)
    y=x-(gain/Ts);
elseif v<=(-tol)
    y=x-(gain/Ts);
elseif v>tol;
    y=x+(gain/Ts);
else
    y=0;
end

== matlab function pacificpower360amxt/Pacific Power 360-AMXT/power-3/control_power-3/conrol/MATLAB Function2 ==
  data: t input; y output; Vrms input; F input; theta1 input
function y = fcn(t,Vrms,F,theta1)
y = sqrt(2)*Vrms*sin(2*pi*F*t + theta1*pi/180);
